simulink model "observer_test"  (R2014b)
settings: Solver=ode45  StartTime=0.0  StopTime=10.0  RelTol=1e-3
values from neighbouring files (symbols this model uses):
  A11 = A2(1,1)    [zad_8.m]
  A12 = A2(1,2:3)    [zad_8.m]
  A21 = A2(2:3,1)    [zad_8.m]
  A22 = A2(2:3,2:3)    [zad_8.m]
  B_1 = B2(1,1)    [zad_8.m]
  B_2 = B2(2:3,1)    [zad_8.m]
  L = acker(A22',A12', [z2(kz2) z3(kz3)])'    [zad_8.m]
  x0_observer = [ 0 0 ]    [zad_8.m]
undefined symbols (not defined in the file or in its folder): A2, B2, K, Tp, x0
settings Model: Creator=Konrad  LastModifiedBy=Konrad

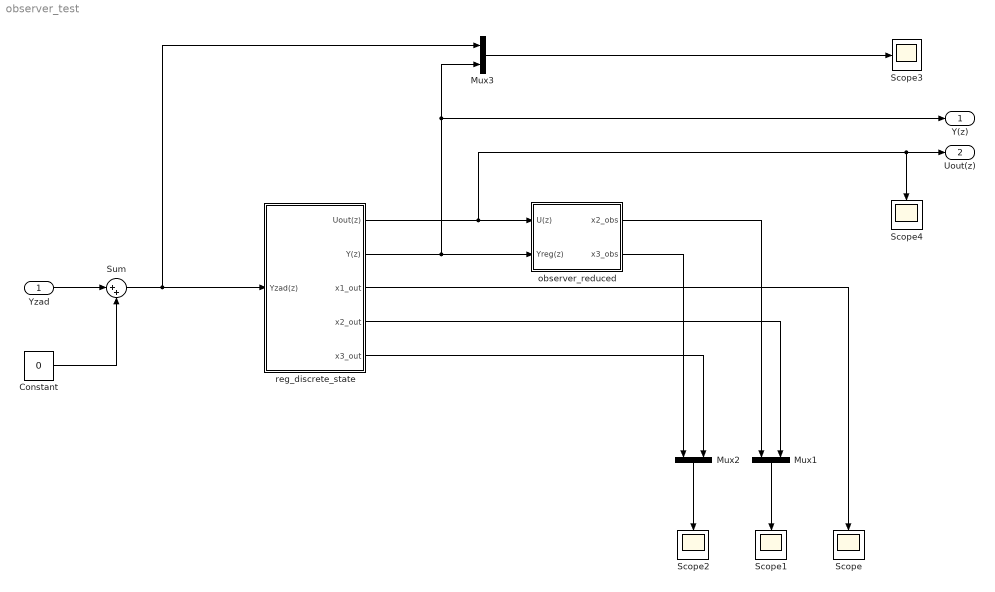
== system observer_test ==
  Yzad : Inport
  Constant : Constant  Value=0
  Mux1 : Mux  Inputs=2
  Mux2 : Mux  Inputs=2
  Mux3 : Mux  Inputs=2
  Scope{,1..4} (5 alike) : Scope
      Scope2 settings: SaveName=ScopeData2
      Scope3 settings: SaveName=ScopeData3
      Scope4 settings: SaveName=ScopeData4
  Sum : Sum  Inputs=|++
  observer_reduced : Subsystem
  reg_discrete_state : Subsystem
  Y(z) : Outport
  Uout(z) : Outport  Port=2
  wires:
  Mux1/1 -> Scope1/1
  Mux2/1 -> Scope2/1
  reg_discrete_state/4(x2_out) -> Mux1/2
  reg_discrete_state/5(x3_out) -> Mux2/2
  reg_discrete_state/3(x1_out) -> Scope/1
  Constant/1 -> Sum/2
  reg_discrete_state/1(Uout(z)) -> Scope4/1, Uout(z)/1, observer_reduced/1(U(z))
  observer_reduced/2(x3_obs) -> Mux2/1
  observer_reduced/1(x2_obs) -> Mux1/1
  reg_discrete_state/2(Y(z)) -> Mux3/2, Y(z)/1, observer_reduced/2(Yreg(z))
  Sum/1 -> Mux3/1, reg_discrete_state/1(Yzad(z))
  Yzad/1 -> Sum/1
  Mux3/1 -> Scope3/1

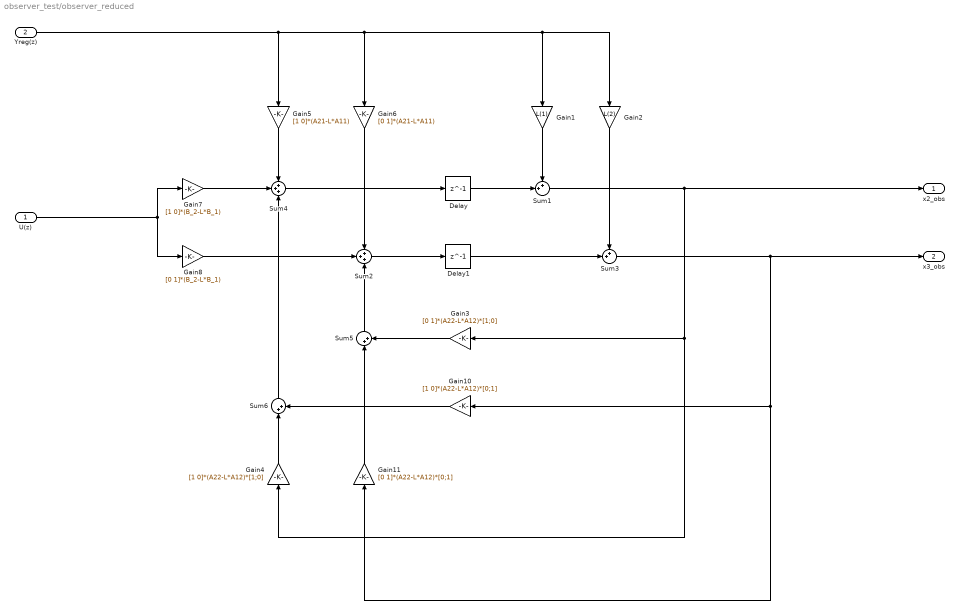
== system observer_test/observer_reduced ==
  U(z) : Inport
  Yreg(z) : Inport  Port=2
  Delay : Delay  DelayLength=1  InitialCondition=x0_observer(1)  SampleTime=Tp
  Delay1 : Delay  DelayLength=1  InitialCondition=x0_observer(2)  SampleTime=Tp
  Gain1 : Gain  Gain=L(1)
  Gain10 : Gain  Gain=[1 0]*(A22-L*A12)*[0;1]
  Gain11 : Gain  Gain=[0 1]*(A22-L*A12)*[0;1]
  Gain2 : Gain  Gain=L(2)
  Gain3 : Gain  Gain=[0 1]*(A22-L*A12)*[1;0]
  Gain4 : Gain  Gain=[1 0]*(A22-L*A12)*[1;0]
  Gain5 : Gain  Gain=[1 0]*(A21-L*A11)
  Gain6 : Gain  Gain=[0 1]*(A21-L*A11)
  Gain7 : Gain  Gain=[1 0]*(B_2-L*B_1)
  Gain8 : Gain  Gain=[0 1]*(B_2-L*B_1)
  Sum1 : Sum  Inputs=++|
  Sum2 : Sum  Inputs=+++
  Sum3 : Sum  Inputs=++|
  Sum4 : Sum  Inputs=+++
  Sum5 : Sum  Inputs=|++
  Sum6 : Sum  Inputs=|++
  x2_obs : Outport
  x3_obs : Outport  Port=2
  wires:
  Gain4/1 -> Sum6/1
  U(z)/1 -> Gain7/1, Gain8/1
  Sum3/1 -> x3_obs/1, Gain11/1, Gain10/1
  Gain1/1 -> Sum1/1
  Delay/1 -> Sum1/2
  Gain5/1 -> Sum4/1
  Sum1/1 -> x2_obs/1, Gain4/1, Gain3/1
  Gain11/1 -> Sum5/1
  Gain7/1 -> Sum4/2
  Sum4/1 -> Delay/1
  Gain2/1 -> Sum3/1
  Sum6/1 -> Sum4/3
  Gain3/1 -> Sum5/2
  Delay1/1 -> Sum3/2
  Yreg(z)/1 -> Gain2/1, Gain1/1, Gain6/1, Gain5/1
  Gain10/1 -> Sum6/2
  Sum2/1 -> Delay1/1
  Gain8/1 -> Sum2/2
  Gain6/1 -> Sum2/1
  Sum5/1 -> Sum2/3

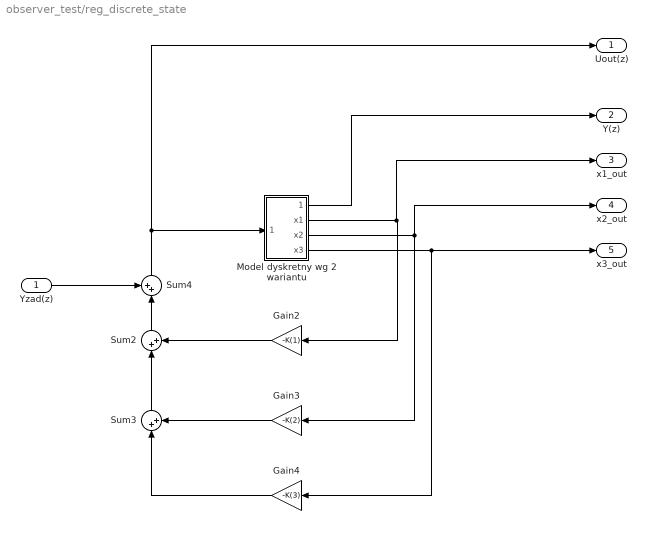
== system observer_test/reg_discrete_state ==
  Yzad(z) : Inport
  Gain2 : Gain  Gain=-K(1)
  Gain3 : Gain  Gain=-K(2)
  Gain4 : Gain  Gain=-K(3)
  Model dyskretny wg 2 wariantu : Subsystem
  Sum2 : Sum  Inputs=|++
  Sum3 : Sum  Inputs=|++
  Sum4 : Sum  Inputs=++|
  Uout(z) : Outport
  Y(z) : Outport  Port=2
  x1_out : Outport  Port=3
  x2_out : Outport  Port=4
  x3_out : Outport  Port=5
  wires:
  Gain2/1 -> Sum2/2
  Gain3/1 -> Sum3/2
  Gain4/1 -> Sum3/1
  Sum3/1 -> Sum2/1
  Sum2/1 -> Sum4/2
  Yzad(z)/1 -> Sum4/1
  Model dyskretny wg 2 wariantu/1(Y(z)) -> Y(z)/1
  Model dyskretny wg 2 wariantu/2(x1) -> x1_out/1, Gain2/1
  Model dyskretny wg 2 wariantu/4(x3) -> Gain4/1, x3_out/1
  Model dyskretny wg 2 wariantu/3(x2) -> Gain3/1, x2_out/1
  Sum4/1 -> Uout(z)/1, Model dyskretny wg 2 wariantu/1(U(z))

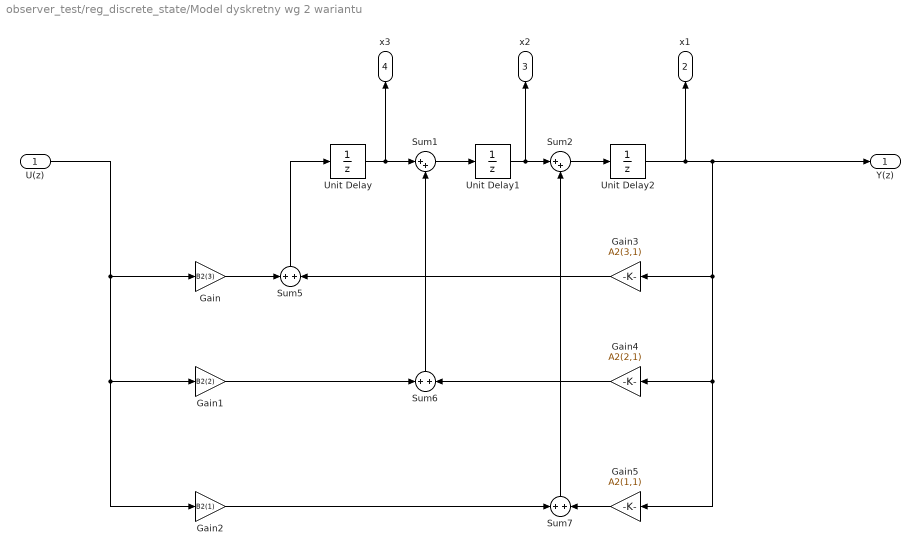
== system observer_test/reg_discrete_state/Model dyskretny wg 2 wariantu ==
  U(z) : Inport
  Gain : Gain  Gain=B2(3)
  Gain1 : Gain  Gain=B2(2)
  Gain2 : Gain  Gain=B2(1)
  Gain3 : Gain  Gain=A2(3,1)
  Gain4 : Gain  Gain=A2(2,1)
  Gain5 : Gain  Gain=A2(1,1)
  Sum1 : Sum  Inputs=|++
  Sum2 : Sum  Inputs=|++
  Sum5 : Sum  Inputs=+|+
  Sum6 : Sum  Inputs=+|+
  Sum7 : Sum  Inputs=+|+
  Unit Delay : UnitDelay  InitialCondition=x0(3)  SampleTime=Tp
  Unit Delay1 : UnitDelay  InitialCondition=x0(2)  SampleTime=Tp
  Unit Delay2 : UnitDelay  InitialCondition=x0(1)  SampleTime=Tp
  Y(z) : Outport
  x1 : Outport  Port=2
  x2 : Outport  Port=3
  x3 : Outport  Port=4
  wires:
  Sum1/1 -> Unit Delay1/1
  Unit Delay1/1 -> x2/1, Sum2/1
  Sum2/1 -> Unit Delay2/1
  Unit Delay/1 -> x3/1, Sum1/1
  Gain1/1 -> Sum6/1
  Gain4/1 -> Sum6/2
  Unit Delay2/1 -> x1/1, Y(z)/1, Gain3/1, Gain4/1, Gain5/1
  Gain3/1 -> Sum5/2
  Gain/1 -> Sum5/1
  Gain5/1 -> Sum7/2
  Sum7/1 -> Sum2/2
  Sum5/1 -> Unit Delay/1
  Gain2/1 -> Sum7/1
  Sum6/1 -> Sum1/2
  U(z)/1 -> Gain/1, Gain1/1, Gain2/1
